simulink model "model_affc"  (R2016b)
settings: Solver=FixedStepDiscrete  StartTime=0.0  StopTime=inf  FixedStep=sampleTime  RelTol=1e-3
PostLoadFcn:
  | model_affc_parameters;
InitFcn:
  | model_affc_parameters;
StartFcn:
  | model_affc_parameters;
values from neighbouring files (symbols this model uses):
  Lb = 0.07    [model_affc_parameters.m]    (also in parameters_sysid.m; parameters_sysid_admittance.m)
  Lf = 0.238    [model_affc_parameters.m]    (also in parameters_sysid.m; parameters_sysid_admittance.m)
  Lu = 0.153    [model_affc_parameters.m]    (also in parameters_sysid.m; parameters_sysid_admittance.m)
  sampleTime = 0.001    [model_affc_parameters.m]    (also in parameters_sysid.m; parameters_sysid_admittance.m)
undefined symbols (not defined in the file or in its folder): FM1
libraries: simulink x14, LibraryFM x14
(part 2 of 2)

== matlab function model_affc/Robot1/DataToEtherCAT/FTSensorError/MATLAB Function ==
  data: ForcesTorques input; e output; MaxForcesTorques input
function e = fcn(ForcesTorques, MaxForcesTorques)

% throw error when any of the forces/torques go over a max allowable value
if any(abs(ForcesTorques) > MaxForcesTorques) 
    e = 1;
else
    e = 0;
end

== matlab function model_affc/Robot1/Controller_PD/PD + AFFC/AFFC/AFFC ==
  data: p output; t input; q input; qdot input; qddot input; e input; tau output; Lf parameter; Lu parameter; Lb parameter; w input
function [p,tau] = affc(t, q, qdot, qddot, e, Lf, Lu, Lb,w)

persistent p_;

if isempty(p_)
%     p_ = [0.00173;0.00159;0.048;0.07889;-0.00389;0.08784;-0.00474];
    p_ = zeros(7,1);
end


% jacobians
J = func_eq_Je(q(1),q(2),Lf,Lu,Lb);
Jdot = func_eq_Jedot(q(1),q(2),qdot(1),qdot(2),Lf,Lu,Lb);

% create Psi
Psi = [diag([qddot(1) qddot(2)]) J'*J*qddot+J'*Jdot*qdot [sign(qdot(1)) qdot(1); 0 0] [0 0;sign(qdot(2)) qdot(2)] ];

% learning matrix Gamma
eta = 0.95*exp(-t/150) + 0.05;

wI = w(1);
wme = w(2);
wfd = w(3);
wfs = w(4);

Gamma = eta*diag([wI wI wme wfs wfd wfs wfd]);

% update p (parameter vector)
% learning rule
dp = Gamma*Psi'*e;
p_ = p_ + dp;

% Psi = [diag([qddot(1) qddot(2)]) J'*J*qddot+J'*Jdot*qdot [ssign(qdot(1)) qdot(1); 0 0] [0 0;ssign(qdot(2)) qdot(2)] ];

% feedforward torque
tau = Psi*p_;

p = p_;

function y = ssign(u,beta)
% soft sign
if nargin == 1
    beta = 150;
end

y = 2./(1+exp(-beta*u))-1;

== matlab function model_affc/Robot1/DataFromEtherCAT/Calculate Arrange Joint and Op Space/forward kinematics/Je ==
  data: q input; Je output size=[2 2]; Lf parameter; Lu parameter; Lb parameter
function Je = Je( q, Lf, Lu, Lb)
%#codegen

% Calculate the Jacobian for this particular device configuration.
% Note that the function func_eq_Je needs to be in the libraries/kinematis_functions folder

% jacobians
Je = func_eq_Je(q(1),q(2),Lf,Lu,Lb);

== matlab function model_affc/Robot1/DataFromEtherCAT/Calculate Arrange Joint and Op Space/forward kinematics/Jedot ==
  data: q input; qdot input; Jedot output size=[2 2]; Lf parameter; Lu parameter; Lb parameter
function Jedot = Jedot( q, qdot, Lf, Lu, Lb)
%#codegen

% Calculate the time derivative of the Jacobian for this particular device configuration.
% Note that the function func_eq_Je needs to be in the libraries/kinematis_functions folder


% jacobians
Jedot = func_eq_Jedot(q(1),q(2),qdot(1),qdot(2),Lf,Lu,Lb);

== matlab function model_affc/Robot1/DataFromEtherCAT/FTSensor_K6D27/CorrectOffset ==
  data: u_in input; u_out output; reset input; corrected output
function [u_out,corrected] = CorrectOffset(u_in,reset)
%#codegen

persistent data_ offset_ counter_ corrected_;
N = 1000;

% initialize
if isempty(data_)
    data_ = zeros(size(u_in,1), N);
    offset_ = zeros(size(u_in));
    counter_ = 1;
    corrected_ = 0;
end

if (counter_ <= N)
    data_(:,counter_) = u_in;
end

counter_ = counter_ + 1;
if reset
    counter_ = 1;
end

% calculate mean
if counter_ == N
    corrected_ = 1;
    offset_ = mean(data_,2);
end

corrected = corrected_;
u_out = u_in - offset_;

== matlab function model_affc/Robot1/DataFromEtherCAT/Calculate Arrange Joint and Op Space/IK all joints ==
  data: x input; q_all output; Lf parameter; Lu parameter; Lb parameter
function q_all = IK_all(x,Lf,Lu,Lb)
%#codegen

q_all = func_eqs_IK_all(x(1),x(2),Lf,Lu,Lb);

if any(isnan(q_all)) || any(isinf(q_all))
    q_all = zeros(5,1);
end

== matlab function model_affc/Robot1/DataFromEtherCAT/Calculate Arrange Joint and Op Space/forward kinematics/calculate xddot ==
  data: qddot input; qdot input size=[2 1]; J input; xddot output size=[2 1]; Jdot input
function xddot = calc_xddot(qddot, qdot, J, Jdot)
%#codegen

xddot = J*qddot + Jdot*qdot;

== matlab function model_affc/Robot1/DataToEtherCAT/CreateSingleErrorValue2/ErrorToPower2 ==
  data: u input; e output
function e = errorToPowerOf2(u)

e = (2.^(0:length(u)-1))*u;

== matlab function model_affc/Robot1/DataToEtherCAT/CreateSingleErrorValue1/ErrorToPower2 ==
  data: u input; e output
function e = errorToPowerOf2(u)

e = (2.^(0:length(u)-1))*u;

== matlab function model_affc/Robot1/DataFromEtherCAT/FTSensor_K6D27/SensorToOperationalSpace ==
  data: q_all input; Fs input; FTOpSpace output; transmatside input
function FTOpSpace = ForceSensorToOperationalSpace(q_all,Fs,transmatside)
%#codegen
q1 = q_all(1);
q2 = q_all(2);
q4 = q_all(4);
q5 = q_all(5);

% based on which arm the force sensor is connected
switch transmatside
    case 1
        alpha = pi-q2;   
        beta = q1+alpha-pi/2;
        R0 = rotmat(beta);
        R = blkdiag(R0,R0); % transform forces and moments
    case 2
        alpha = -(pi - q4);
        beta = q5+alpha-pi/2;
        R0 = rotmat(beta);
        R = blkdiag(R0,R0); % transform forces and moments
    otherwise
        R = eye(length(Fs));
end

% transform force
FTOpSpace = R*Fs;

function R = rotmat(q)

R = [cos(q) -sin(q) 0;...
      sin(q)  cos(q) 0;...
      0       0      1];

== matlab function model_affc/Robot1/DataToEtherCAT/WorkspacePositionGuard/CheckInternalAngles ==
  data: theta input; angleError output
function angleError = checkInternalErrors(theta)
%#codegen


angleError = 0;
if any(theta([2 4]) >= 0.95*pi)
    angleError = 1;
end

== matlab function model_affc/Robot1/DataToEtherCAT/WorkspacePositionGuard/EndpointPositionGuard ==
  data: correctState input; xe input; error output
function error = fcn(correctState, xe)
%#codegen


error = 0;

% only check workspace boundaries after homing state is done
if ~correctState 
    return; 
end

% x0 = 0;
% y0 = 0.2354;
% a = 0.11;
% b = 0.08;

% workspace (see design document)
x0 = 0;
y0 = 0.25024;
a = 0.1746;
b = 0.13;%0.1048;

% check if endpoint is outside a predefined ellipse
x = xe(1);
y = xe(2);

% workspace is defined as an ellipse
e = (x-x0)^2 / a^2 + (y-y0)^2 / b^2;

% if is larger than 1, the endpoint is outside the workspace
if e > 1
    error = 1;
end
